simulink model "solution_basicOperations_exercise"  (R2021a)
settings: Solver=VariableStepAuto  StartTime=0.0  StopTime=10.0  RelTol=1e-3
libraries: visiongeotforms x2, visionsources x1
settings Model: Creator=lipingw  LastModifiedBy=mmordeka
settings SolverCC: AlgebraicLoopSolver=TrustRegion
settings DebuggingCC: SFMachineParentedDataDiag=warning

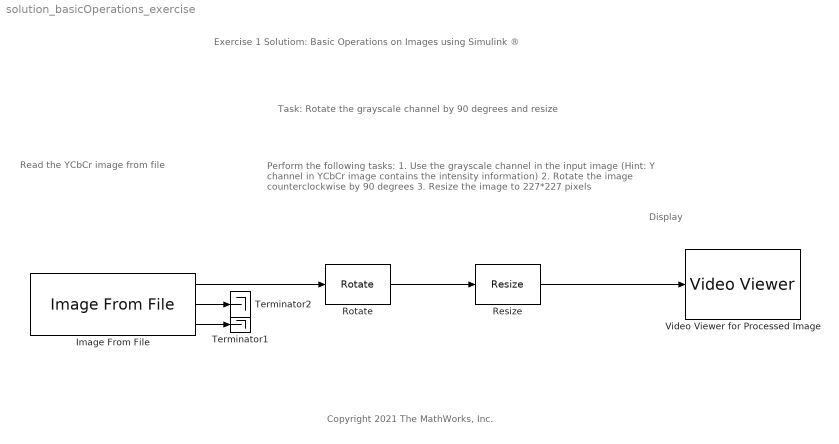
== system solution_basicOperations_exercise ==
  note: Task: Rotate the grayscale channel by 90 degrees and resize
  note: Copyright 2021 The MathWorks, Inc.
  note: Exercise 1 Solutiom: Basic Operations on Images using Simulink ®
  note: Display
  note: Perform the following tasks:
      | 1. Use the grayscale channel in the input image
      | (Hint: Y channel in YCbCr image contains the intensity information)
      | 2. Rotate the image counterclockwise by 90 degrees
      | 3. Resize the image to 227*227 pixels
  note: Read the YCbCr image from file
  Image From File : visionsources/Image From File  Tag=vipblks_nd  FileName=droneYcbcr.jpg  Ts=inf  imagePorts=Separate color signals  OutPortLabels=Y|Cb|Cr  ImageDataType=Inherit from input image  sdImageDataType=uint(8)  Signed=on  WordLength=16  FractionLengthMode=User-defined  FractionLength=15
  Resize : visiongeotforms/Resize  specify=Output size as a percentage of input size  rfactor=[227 227]  outCols=25  outRows=25  outRowsCols=[25 35]  interp_method=Bilinear  antialias=on  useROI=off  roiFlag=off  roundingMode=Nearest  overflowMode=on  prodOutputMode=Binary point scaling  prodOutputWordLength=32  prodOutputFracLength=10
      settings: SourceProductBaseCode=VP
  Rotate : visiongeotforms/Rotate  outSizeR=Expanded to fit rotated input image  src_angle=Specify via dialog  unit_angle=Degrees  angle=pi/2  maxAngle=pi  dispImage=Top-left corner  method=Table lookup  fillVal=0  interpMethod=Bilinear  roundingMode=Nearest  overflowMode=on  prodOutputMode=Binary point scaling  prodOutputWordLength=32  prodOutputFracLength=10
  Terminator1 : Terminator
  Terminator2 : Terminator
  Video Viewer for Processed Image : VideoViewer  FigPos=[2725 1237 802 628]
  wires:
  Image From File/2 -> Terminator2/1
  Image From File/3 -> Terminator1/1
  Image From File/1 -> Rotate/1
  Rotate/1 -> Resize/1
  Resize/1 -> Video Viewer for Processed Image/1
